simulink model "schemasimulink"  (R2023b)
settings: Solver=VariableStepAuto  StartTime=0.0  StopTime=10.0  RelTol=1e-3
values from neighbouring files (symbols this model uses):
  A = sys_pade.A    [attempt.m]    (also in model_approximation.m; observer.m = [-7.9641 0 8.7857; 1.0000 0 0; 0 0 -35.1427]; progetto.m = [0 1; 0 -1/Tm]; tuning.m)
  B = sys_pade.B    [attempt.m]    (also in model_approximation.m; observer.m = [-1;0;8]; progetto.m = [0 ;km/Tm]; tuning.m)
  K = K_tilde(1:3)    [freq_closed_loop.m]
  r = 50    [progetto.m]
settings Model: Creator=giova  LastModifiedBy=giova

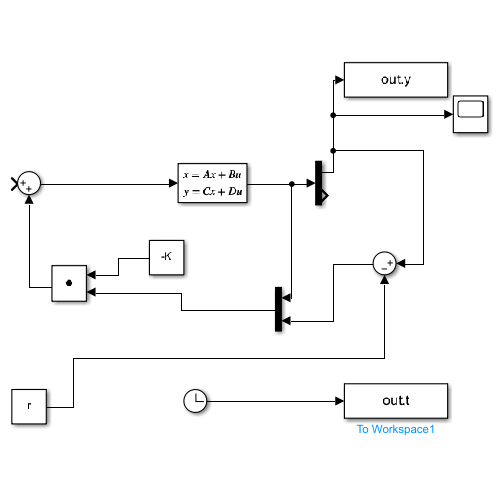
[thumbnail: Simulink's stored preview of the top-level diagram]
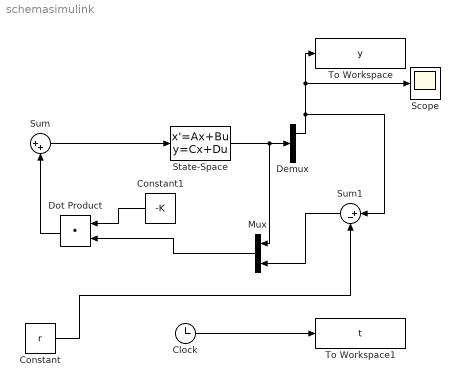
== system schemasimulink ==
  Clock : Clock
  Constant : Constant  Value=r
  Constant1 : Constant  Value=-K
  Demux : Demux  Outputs=2
  Dot Product : DotProduct  OutDataTypeStr=Inherit: Inherit via internal rule
  Mux : Mux  Inputs=2
  Scope : Scope
  State-Space : StateSpace  A=A  B=B  C=eye(2)  D=[0; 0]  InitialCondition=0
  Sum : Sum  Inputs=|++
  Sum1 : Sum  Inputs=|+-
  To Workspace : ToWorkspace  VariableName=y  SampleTime=-1
  To Workspace1 : ToWorkspace  VariableName=t  SampleTime=-1
  wires:
  State-Space/1 -> Mux/1, Demux/1
  Clock/1 -> To Workspace1/1
  Demux/1 -> Sum1/1, Scope/1, To Workspace/1
  Constant/1 -> Sum1/2
  Sum/1 -> State-Space/1
  Sum1/1 -> Mux/2
  Mux/1 -> Dot Product/2
  Constant1/1 -> Dot Product/1
  Dot Product/1 -> Sum/2
